simulink model "PTBatteryCU"  (R2022b)
settings: Solver=ode45  StartTime=0.0  StopTime=inf  RelTol=1e-3  EnableMultiTasking=on
(part 3 of 3)

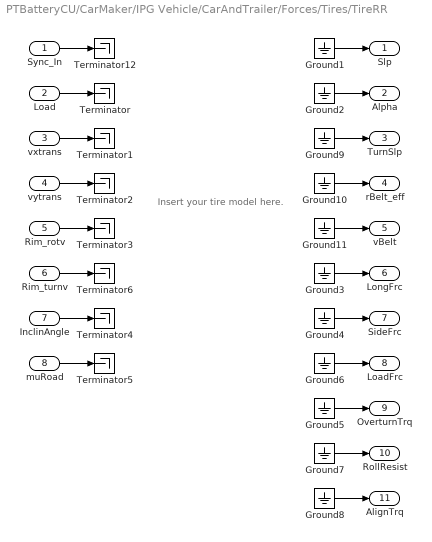
== system PTBatteryCU/CarMaker/IPG Vehicle/CarAndTrailer/Forces/Tires/TireRR ==
  note: Insert your tire model here.
  Sync_In : Inport
  Load : Inport  Port=2
  vxtrans : Inport  Port=3
  vytrans : Inport  Port=4
  Rim_rotv : Inport  Port=5
  Rim_turnv : Inport  Port=6
  InclinAngle : Inport  Port=7
  muRoad : Inport  Port=8
  Ground{1..11} (11 alike) : Ground
  Terminator{,1..6,12} (8 alike) : Terminator
  Slp : Outport  VectorParamsAs1DForOutWhenUnconnected=off
  Alpha : Outport  Port=2  VectorParamsAs1DForOutWhenUnconnected=off
  TurnSlp : Outport  Port=3  VectorParamsAs1DForOutWhenUnconnected=off
  rBelt_eff : Outport  Port=4  VectorParamsAs1DForOutWhenUnconnected=off
  vBelt : Outport  Port=5  VectorParamsAs1DForOutWhenUnconnected=off
  LongFrc : Outport  Port=6  VectorParamsAs1DForOutWhenUnconnected=off
  SideFrc : Outport  Port=7  VectorParamsAs1DForOutWhenUnconnected=off
  LoadFrc : Outport  Port=8  VectorParamsAs1DForOutWhenUnconnected=off
  OverturnTrq : Outport  Port=9  VectorParamsAs1DForOutWhenUnconnected=off
  RollResist : Outport  Port=10  VectorParamsAs1DForOutWhenUnconnected=off
  AlignTrq : Outport  Port=11  VectorParamsAs1DForOutWhenUnconnected=off
  wires:
  Ground11/1 -> vBelt/1
  Ground10/1 -> rBelt_eff/1
  Ground9/1 -> TurnSlp/1
  Rim_turnv/1 -> Terminator6/1
  Sync_In/1 -> Terminator12/1
  Ground2/1 -> Alpha/1
  Ground3/1 -> LongFrc/1
  Ground4/1 -> SideFrc/1
  Ground5/1 -> OverturnTrq/1
  vxtrans/1 -> Terminator1/1
  vytrans/1 -> Terminator2/1
  Rim_rotv/1 -> Terminator3/1
  InclinAngle/1 -> Terminator4/1
  muRoad/1 -> Terminator5/1
  Load/1 -> Terminator/1
  Ground1/1 -> Slp/1
  Ground6/1 -> LoadFrc/1
  Ground7/1 -> RollResist/1
  Ground8/1 -> AlignTrq/1

== system PTBatteryCU/CarMaker/IPG Vehicle/PowerTrain/BCU Example/MyBatteryCU/If Ignition ==
  BattLV.AOC : Inport
  Capacity_LV : Inport  Port=2
  Pwr_HV1toLV_trg Input : Inport  Port=3
  Ignition : ActionPort  ActionPortLabel=else
  Bus Creator : BusCreator  Inputs=3
  Constant : Constant  Value=100.0
  Divide : Product  Inputs=*/
  Gain : Gain  Gain=100
  out : Outport  InitialOutput=[,100,]  VectorParamsAs1DForOutWhenUnconnected=off
  wires:
  Bus Creator/1 -> out/1
  Pwr_HV1toLV_trg Input/1 -> Bus Creator/3  "Pwr_HV1toLV_trg"
  Gain/1 -> Bus Creator/1  "SOC_LV"
  Divide/1 -> Gain/1
  Capacity_LV/1 -> Divide/2
  BattLV.AOC/1 -> Divide/1
  Constant/1 -> Bus Creator/2  "SOH_LV"

== system PTBatteryCU/CarMaker/IPG Vehicle/PowerTrain/BCU Example/MyBatteryCU/If Ignition1 ==
  BattHV.AOC : Inport
  Capacity_HV : Inport  Port=2
  Ignition : ActionPort  ActionPortLabel=else
  Bus Creator : BusCreator  Inputs=2
  Constant : Constant  Value=100.0
  Divide : Product  Inputs=*/
  Gain : Gain  Gain=100
  out : Outport  InitialOutput=[,100,]  VectorParamsAs1DForOutWhenUnconnected=off
  wires:
  Bus Creator/1 -> out/1
  Gain/1 -> Bus Creator/1  "SOC_HV"
  Divide/1 -> Gain/1
  Capacity_HV/1 -> Divide/2
  BattHV.AOC/1 -> Divide/1
  Constant/1 -> Bus Creator/2  "SOH_HV"

== system PTBatteryCU/CarMaker/IPG Vehicle/PowerTrain/BCU Example/MyBatteryCU/If no Ignition ==
  no Ignition : ActionPort  ActionPortLabel=if(~u1)
  Bus Creator : BusCreator  Inputs=3
  Constant : Constant  Value=0.0
  Constant1 : Constant  Value=0.0
  Constant2 : Constant  Value=0.0
  out : Outport  InitialOutput=0  VectorParamsAs1DForOutWhenUnconnected=off
  wires:
  Bus Creator/1 -> out/1
  Constant2/1 -> Bus Creator/3  "Pwr_HV1toLV_trg"
  Constant/1 -> Bus Creator/1  "SOC_LV"
  Constant1/1 -> Bus Creator/2  "SOH_LV"

== system PTBatteryCU/CarMaker/IPG Vehicle/PowerTrain/BCU Example/MyBatteryCU/If no Ignition1 ==
  no Ignition : ActionPort  ActionPortLabel=if(~u1)
  Bus Creator : BusCreator  Inputs=2
  Constant : Constant  Value=0.0
  Constant1 : Constant  Value=0.0
  out : Outport  InitialOutput=0  VectorParamsAs1DForOutWhenUnconnected=off
  wires:
  Bus Creator/1 -> out/1
  Constant/1 -> Bus Creator/1  "SOC_HV"
  Constant1/1 -> Bus Creator/2  "SOH_HV"

== system PTBatteryCU/CarMaker/IPG Vehicle/PowerTrain/BCU Example/PTBatteryCU_In/CreateBus BCU BattHV ==
  In : Inport
  BusCreator : BusCreator  Inputs=8
  Demux : Demux  Outputs=8
      settings: DisplayOption=none
  Out : Outport  VectorParamsAs1DForOutWhenUnconnected=off
  wires:
  Demux/3 -> BusCreator/3  "BCU BattHV Energy"
  Demux/2 -> BusCreator/2  "BCU BattHV AOC"
  Demux/4 -> BusCreator/4  "BCU BattHV Pwr_max"
  BusCreator/1 -> Out/1
  Demux/6 -> BusCreator/6  "BCU BattHV TempCool_out"
  Demux/5 -> BusCreator/5  "BCU BattHV Temp"
  Demux/1 -> BusCreator/1  "BCU BattHV Current"
  In/1 -> Demux/1
  Demux/7 -> BusCreator/7  "BCU BattHV Temp_trg"
  Demux/8 -> BusCreator/8  "BCU BattHV MassFlowCool_trg"

== system PTBatteryCU/CarMaker/IPG Vehicle/PowerTrain/BCU Example/PTBatteryCU_In/CreateBus BCU BattLV ==
  In : Inport
  BusCreator : BusCreator  Inputs=8
  Demux : Demux  Outputs=8
      settings: DisplayOption=none
  Out : Outport  VectorParamsAs1DForOutWhenUnconnected=off
  wires:
  Demux/5 -> BusCreator/5  "BCU BattLV Temp"
  Demux/4 -> BusCreator/4  "BCU BattLV Pwr_max"
  In/1 -> Demux/1
  Demux/3 -> BusCreator/3  "BCU BattLV Energy"
  BusCreator/1 -> Out/1
  Demux/1 -> BusCreator/1  "BCU BattLV Current"
  Demux/2 -> BusCreator/2  "BCU BattLV AOC"
  Demux/6 -> BusCreator/6  "BCU BattLV TempCool_out"
  Demux/7 -> BusCreator/7  "BCU BattLV Temp_trg"
  Demux/8 -> BusCreator/8  "BCU BattLV MassFlowCool_trg"

== system PTBatteryCU/CarMaker/IPG Vehicle/PowerTrain/BCU Example/PTBatteryCU_In/CreateBus BCU Input ==
  In : Inport
  BusCreator : BusCreator  Inputs=14
  Demux : Demux  Outputs=14
      settings: DisplayOption=none
  Out : Outport  VectorParamsAs1DForOutWhenUnconnected=off
  wires:
  Demux/14 -> BusCreator/14  "BCU Eta_HV1toHV2"
  Demux/10 -> BusCreator/10  "BCU Pwr_HV1toHV2"
  Demux/9 -> BusCreator/9  "BCU Pwr_HV1toLV"
  Demux/1 -> BusCreator/1  "BCU Ignition"
  Demux/2 -> BusCreator/2  "BCU Pwr_LV"
  BusCreator/1 -> Out/1
  Demux/11 -> BusCreator/11  "BCU Pwr_HV1toLV_max"
  Demux/6 -> BusCreator/6  "BCU Voltage_HV1"
  Demux/8 -> BusCreator/8  "BCU Pwr_HV1toLV_trg"
  In/1 -> Demux/1
  Demux/3 -> BusCreator/3  "BCU Pwr_HV1"
  Demux/12 -> BusCreator/12  "BCU Pwr_HV1toHV2_max"
  Demux/4 -> BusCreator/4  "BCU Pwr_HV2"
  Demux/5 -> BusCreator/5  "BCU Voltage_LV"
  Demux/13 -> BusCreator/13  "BCU Eta_HV1toLV"
  Demux/7 -> BusCreator/7  "BCU Voltage_HV2"

== system PTBatteryCU/CarMaker/IPG Vehicle/PowerTrain/BCU Example/PTBatteryCU_In/CreateBus BCU_Cfg BattHV ==
  In : Inport
  BusCreator : BusCreator  Inputs=6
  Demux : Demux  Outputs=6
      settings: DisplayOption=none
  Out : Outport  VectorParamsAs1DForOutWhenUnconnected=off
  wires:
  BusCreator/1 -> Out/1
  Demux/5 -> BusCreator/5  "BCU_Cfg BattHV Temp_init"
  Demux/1 -> BusCreator/1  "BCU_Cfg BattHV SOC_min"
  Demux/6 -> BusCreator/6  "BCU_Cfg BattHV TempCool_init"
  Demux/4 -> BusCreator/4  "BCU_Cfg BattHV Voltage"
  In/1 -> Demux/1
  Demux/2 -> BusCreator/2  "BCU_Cfg BattHV SOC_max"
  Demux/3 -> BusCreator/3  "BCU_Cfg BattHV Capacity"

== system PTBatteryCU/CarMaker/IPG Vehicle/PowerTrain/BCU Example/PTBatteryCU_In/CreateBus BCU_Cfg BattLV ==
  In : Inport
  BusCreator : BusCreator  Inputs=6
  Demux : Demux  Outputs=6
      settings: DisplayOption=none
  Out : Outport  VectorParamsAs1DForOutWhenUnconnected=off
  wires:
  Demux/4 -> BusCreator/4  "BCU_Cfg BattLV Voltage"
  Demux/3 -> BusCreator/3  "BCU_Cfg BattLV Capacity"
  BusCreator/1 -> Out/1
  Demux/1 -> BusCreator/1  "BCU_Cfg BattLV SOC_min"
  In/1 -> Demux/1
  Demux/2 -> BusCreator/2  "BCU_Cfg BattLV SOC_max"
  Demux/5 -> BusCreator/5  "BCU_Cfg BattLV Temp_init"
  Demux/6 -> BusCreator/6  "BCU_Cfg BattLV TempCool_init"
